simulink model "window_copy_one_in_two_out"  (R2019b)
settings: Solver=VariableStepAuto  StartTime=0.0  StopTime=10.0  RelTol=1e-3
libraries: ModelComposer x1
settings Model: Creator=abehbood  LastModifiedBy=abehbood

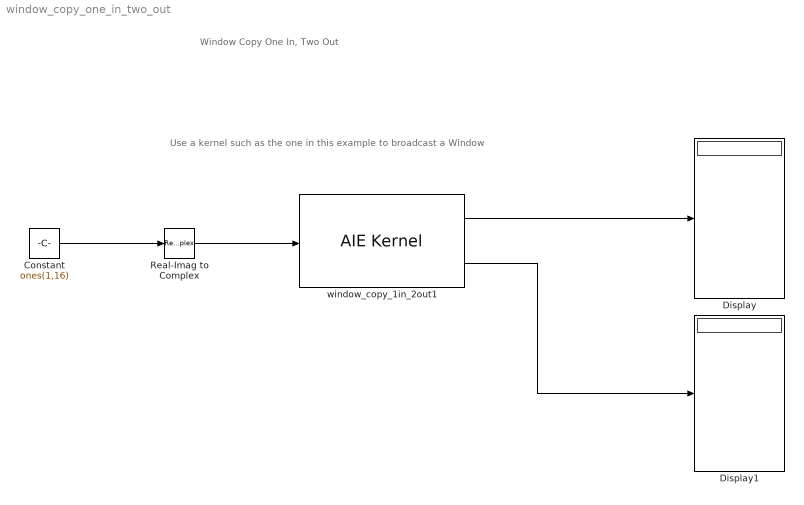
== system window_copy_one_in_two_out ==
  note: Use a kernel such as the one in this example to broadcast a Window
  note: Window Copy
      | One In, Two Out
  Constant : Constant  Value=ones(1,16)  OutDataTypeStr=int16  SampleTime=1
  Display : Display
  Display1 : Display
  Real-Imag to Complex : RealImagToComplex  Input=Real
  window_copy_1in_2out1 : ModelComposer/AIE Kernel  PortAttributesTable={ 'Input', 'cb_in', 'input_window_cint16 * restrict', '16', '0', 'auto', ''; 'Output', 'cb_out0', 'output_window_cint16 * restrict', '16', '', 'auto', ''; 'Output', 'cb_out1', 'output_window_cint16 * restrict', '16', '', 'auto', '' }  PortAttributesEnablement={'off', 'off', 'off', 'on', 'on', 'on', 'off';'off', 'off', 'off', 'on', 'off', 'on', 'off';'off', 'off', 'off', 'on', 'off', 'on', 'off'}  FormalArgDecls={'input_window_cint16 * restrict cb_in', 'output_window_cint16 * restrict cb_out0', 'output_window_cint16 * restrict cb_out1'}  PortWindowSizes={1.600000000000000000e+01; 1.600000000000000000e+01; 1.600000000000000000e+01}  PortWindowMargins={0.000000000000000000e+00; 0.000000000000000000e+00; 0.000000000000000000e+00}  PortSynchronicities={'auto'; 'auto'; 'auto'}  PortSignalSizes={0.000000000000000000e+00; 0.000000000000000000e+00; 0.000000000000000000e+00}  SimLibPath=''  FunctionTabVisible=on  FunctionDescription=void window_copy_1in_2out(input_window_cint16 * restrict cb_in, output_window_cint16 * restrict cb_out0, output_window_cint16 * restrict cb_out1)  KernelHeaderFile=src/kernels/window_copy.h  KernelFunction=window_copy_1in_2out  KernelFunctionSelect=<empty>  KernelSourceFile=src/kernels/window_copy.cc  KernelSearchPaths={'./src/kernels'}  PreProcOptions={}  CoreRuntimeRatio=0.9  KernelLocSpec=off  ColRowLocation=[0 0]
  wires:
  window_copy_1in_2out1/1 -> Display/1
  window_copy_1in_2out1/2 -> Display1/1
  Real-Imag to Complex/1 -> window_copy_1in_2out1/1
  Constant/1 -> Real-Imag to Complex/1
